simulink model "GMCLIB_ClarkInv_BAM_F16"  (Simulink 7.3)
settings: Solver=ode45  StartTime=0.0  StopTime=10.0  RelTol=1e-3
settings Model: Creator=B17364  LastModifiedBy=B17364

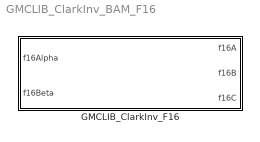
== system GMCLIB_ClarkInv_BAM_F16 ==
  GMCLIB_ClarkInv_F16 : Subsystem  mask(GMCLIB_ClarkInv_F16){}
      mask help: Bit accurate model of inverse Clarke transformation 2ph -> 3ph
      mask init:
      | pos = get_param(gcb, 'Position');width = pos(3) - pos(1); height = pos(4) - pos(2);tX=width/2;tY=height*0.9;
      mask Display: color('black');port_label('input',1,'f16Alpha');port_label('input',2,'f16Beta');port_label('output',1,'f16A');port_label('output',2,'f16B');port_label('output',3,'f16C');color('black');disp('GMCLIB_ClarkInv_F16');color('blue');text(tX,tY, 'BAM', 'horizontalAlignment', 'center');

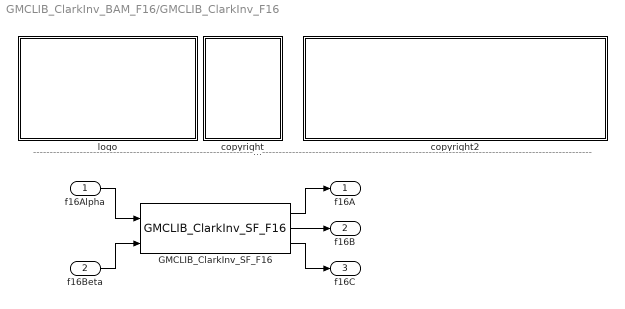
== system GMCLIB_ClarkInv_BAM_F16/GMCLIB_ClarkInv_F16 ==
  note: ---------------------------------------------------------------------------------------------------------------------------------------------------------------------------------------------------
  f16Alpha : Inport  OutDataType=fixdt(1, 16)  OutScaling=2^0
  f16Beta : Inport  Port=2  OutDataType=fixdt(1, 16)  OutScaling=2^0
  GMCLIB_ClarkInv_SF_F16 : S-Function  FunctionName=GMCLIB_ClarkInv_SF_F16  EnableBusSupport=off
  copyright : Subsystem
      mask Display: text(10,90,'FILE:');text(10,75,'DESRIPTION:')text(10,60,'COPYRIGHT:')text(10,45,'VERSION:')text(10,30,'DATE:')
  copyright2 : Subsystem
      mask Display: text(10,90,'GMCLIB_ClarkInv_BAM_F16.mdl');text(10,75,'Inverse Clarke transformation');text(10,60,'Freescale')text(10,45,'0.1');text(10,30,'30-Aug-2011');
  logo : Subsystem
      mask Display: image(imread('logo.jpg'))
  f16A : Outport  OutDataType=fixdt(1, 16)  OutScaling=2^0
  f16B : Outport  Port=2  OutDataType=fixdt(1, 16)  OutScaling=2^0
  f16C : Outport  Port=3  OutDataType=fixdt(1, 16)  OutScaling=2^0
  wires:
  f16Alpha/1 -> GMCLIB_ClarkInv_SF_F16/1
  f16Beta/1 -> GMCLIB_ClarkInv_SF_F16/2
  GMCLIB_ClarkInv_SF_F16/1 -> f16A/1
  GMCLIB_ClarkInv_SF_F16/2 -> f16B/1
  GMCLIB_ClarkInv_SF_F16/3 -> f16C/1

== system GMCLIB_ClarkInv_BAM_F16/GMCLIB_ClarkInv_F16/copyright ==

== system GMCLIB_ClarkInv_BAM_F16/GMCLIB_ClarkInv_F16/copyright2 ==

== system GMCLIB_ClarkInv_BAM_F16/GMCLIB_ClarkInv_F16/logo ==
